simulink model "task_2_2a"  (R2021b)
settings: Solver=VariableStepAuto  StartTime=0.0  StopTime=10  RelTol=1e-3
libraries: simulink x2
settings Model: Creator=osini  LastModifiedBy=osini

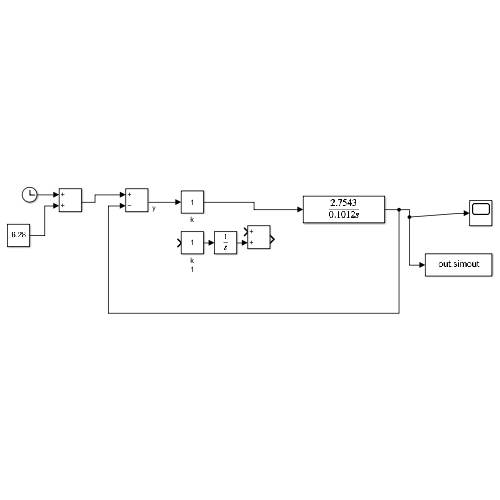
[thumbnail: Simulink's stored preview of the top-level diagram]
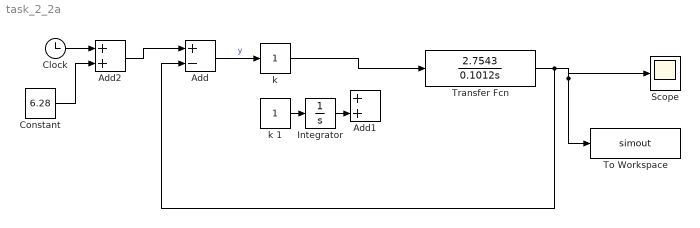
== system task_2_2a ==
  Add : Sum  Inputs=+-
  Add1 : Sum
  Add2 : Sum
  Clock : Clock
  Constant : Constant  Value=6.28
  Integrator : Integrator
  Scope : Scope
  To Workspace : ToWorkspace  VariableName=simout  SaveFormat=Timeseries  SampleTime=-1
  Transfer Fcn : TransferFcn  Numerator=[2.7543]  Denominator="[0.1012  0]"
  "k " : simulink/Math Operations/Slider Gain  gain=1  low=-1000  high=1000
  k 1 : simulink/Math Operations/Slider Gain  gain=1  low=0  high=500
  wires:
  Add/1 -> "k "/1  "y"
  k 1/1 -> Integrator/1
  Integrator/1 -> Add1/2
  Transfer Fcn/1 -> Scope/1, To Workspace/1, Add/2
  Clock/1 -> Add2/1
  Add2/1 -> Add/1
  Constant/1 -> Add2/2
  "k "/1 -> Transfer Fcn/1
